simulink model "VehicleModel2_BusDef"  (R2020b)
settings: Solver=VariableStepAuto  StartTime=0.0  StopTime=10.0  RelTol=1e-3
settings Model: Creator=Authorized User  LastModifiedBy=Authorized User

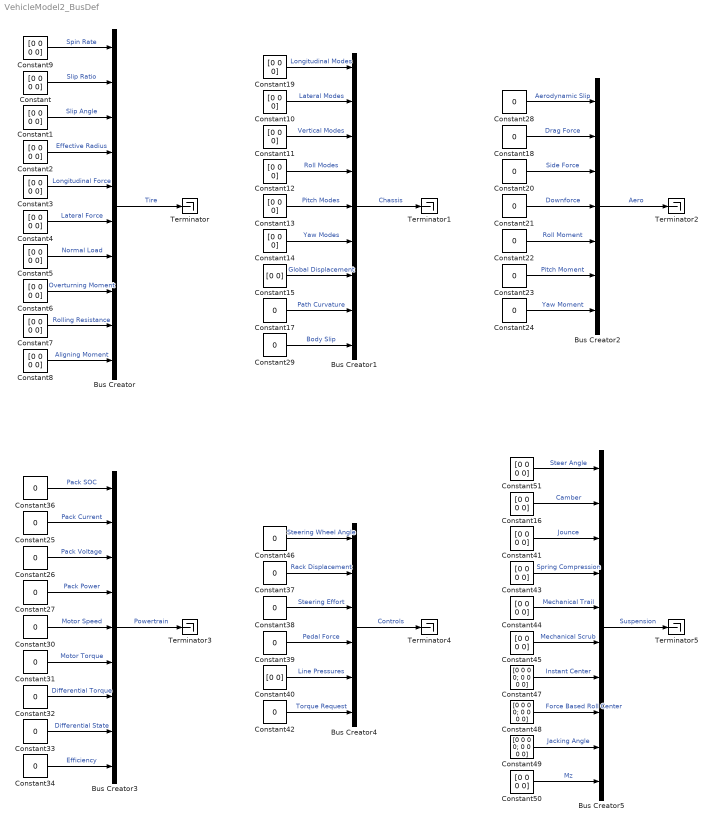
== system VehicleModel2_BusDef ==
  Bus Creator : BusCreator  Inputs=10
  Bus Creator1 : BusCreator  Inputs=9
  Bus Creator2 : BusCreator  Inputs=7
  Bus Creator3 : BusCreator  Inputs=9
  Bus Creator4 : BusCreator  Inputs=6
  Bus Creator5 : BusCreator  Inputs=10
  Constant{,1..9,16,41,43..45,50..51} (17 alike) : Constant  Value=[0 0 0 0]
  Constant{10..14,19} (6 alike) : Constant  Value=[0 0 0]
  Constant15 : Constant  Value=[0 0]
  Constant{17..18,20..34,36..39,42,46} (23 alike) : Constant  Value=0
  Constant40 : Constant  Value=[0 0]
  Constant47 : Constant  Value=[0 0 0 0; 0 0 0 0]
  Constant48 : Constant  Value=[0 0 0 0; 0 0 0 0]
  Constant49 : Constant  Value=[0 0 0 0; 0 0 0 0]
  Terminator{,1..5} (6 alike) : Terminator
  wires:
  Constant/1 -> Bus Creator/2  "Slip Ratio"
  Constant1/1 -> Bus Creator/3  "Slip Angle"
  Constant2/1 -> Bus Creator/4  "Effective Radius"
  Constant3/1 -> Bus Creator/5  "Longitudinal Force"
  Constant4/1 -> Bus Creator/6  "Lateral Force"
  Constant5/1 -> Bus Creator/7  "Normal Load"
  Constant6/1 -> Bus Creator/8  "Overturning Moment"
  Constant7/1 -> Bus Creator/9  "Rolling Resistance"
  Constant8/1 -> Bus Creator/10  "Aligning Moment"
  Constant9/1 -> Bus Creator/1  "Spin Rate"
  Bus Creator/1 -> Terminator/1  "Tire"
  Bus Creator1/1 -> Terminator1/1  "Chassis"
  Constant11/1 -> Bus Creator1/3  "Vertical Modes"
  Constant12/1 -> Bus Creator1/4  "Roll Modes"
  Constant14/1 -> Bus Creator1/6  "Yaw Modes"
  Constant10/1 -> Bus Creator1/2  "Lateral Modes"
  Constant19/1 -> Bus Creator1/1  "Longitudinal Modes"
  Constant13/1 -> Bus Creator1/5  "Pitch Modes"
  Constant15/1 -> Bus Creator1/7  "Global Displacement"
  Bus Creator2/1 -> Terminator2/1  "Aero"
  Constant28/1 -> Bus Creator2/1  "Aerodynamic Slip"
  Constant18/1 -> Bus Creator2/2  "Drag Force"
  Constant20/1 -> Bus Creator2/3  "Side Force"
  Constant21/1 -> Bus Creator2/4  "Downforce"
  Constant22/1 -> Bus Creator2/5  "Roll Moment"
  Constant23/1 -> Bus Creator2/6  "Pitch Moment"
  Constant24/1 -> Bus Creator2/7  "Yaw Moment"
  Bus Creator3/1 -> Terminator3/1  "Powertrain"
  Constant26/1 -> Bus Creator3/3  "Pack Voltage"
  Constant27/1 -> Bus Creator3/4  "Pack Power"
  Constant33/1 -> Bus Creator3/8  "Differential State"
  Constant31/1 -> Bus Creator3/6  "Motor Torque"
  Constant25/1 -> Bus Creator3/2  "Pack Current"
  Constant36/1 -> Bus Creator3/1  "Pack SOC"
  Constant34/1 -> Bus Creator3/9  "Efficiency"
  Constant30/1 -> Bus Creator3/5  "Motor Speed"
  Constant32/1 -> Bus Creator3/7  "Differential Torque"
  Constant38/1 -> Bus Creator4/3  "Steering Effort"
  Bus Creator4/1 -> Terminator4/1  "Controls"
  Constant40/1 -> Bus Creator4/5  "Line Pressures"
  Constant46/1 -> Bus Creator4/1  "Steering Wheel Angle"
  Constant37/1 -> Bus Creator4/2  "Rack Displacement"
  Constant39/1 -> Bus Creator4/4  "Pedal Force"
  Constant17/1 -> Bus Creator1/8  "Path Curvature"
  Constant29/1 -> Bus Creator1/9  "Body Slip"
  Constant42/1 -> Bus Creator4/6  "Torque Request"
  Constant41/1 -> Bus Creator5/3  "Jounce"
  Bus Creator5/1 -> Terminator5/1  "Suspension"
  Constant44/1 -> Bus Creator5/5  "Mechanical Trail"
  Constant48/1 -> Bus Creator5/8  "Force Based Roll Center"
  Constant45/1 -> Bus Creator5/6  "Mechanical Scrub"
  Constant51/1 -> Bus Creator5/1  "Steer Angle"
  Constant47/1 -> Bus Creator5/7  "Instant Center"
  Constant16/1 -> Bus Creator5/2  "Camber"
  Constant43/1 -> Bus Creator5/4  "Spring Compression"
  Constant49/1 -> Bus Creator5/9  "Jacking Angle"
  Constant50/1 -> Bus Creator5/10  "Mz"
